simulink model "SRRC_Cosimulation"  (R2016a)
settings: Solver=ode3  StartTime=0.0  StopTime=0.5  RelTol=1e-3
undefined symbols (not defined in the file or in its folder): image, port_label
libraries: aldec_ahdl x2, dspsrcs4 x2
settings Model: Creator=Sara  LastModifiedBy=paolosassi
settings DataIOCC: LimitDataPoints=on  SaveFormat=Array
settings HardwareCC: ProdBitPerPointer=32  ProdLargestAtomicFloat=None  ProdIntDivRoundTo=Undefined  ProdEndianess=Unspecified  ProdWordSize=32  ProdHWDeviceType=32-bit Generic
settings ModelReferenceCC: PropagateSignalLabelsOutOfModel=off
settings ConfigComp: CovModelRefEnable=Off

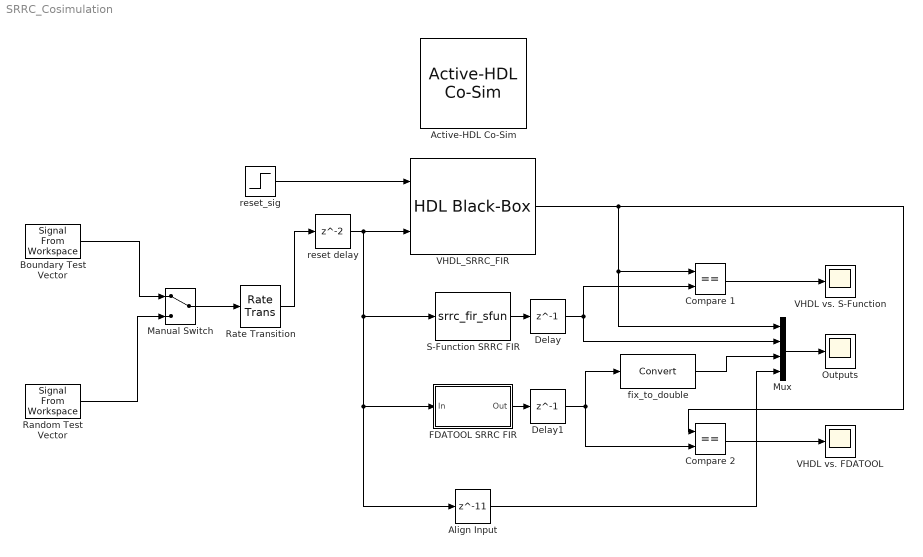
== system SRRC_Cosimulation ==
  Active-HDL Co-Sim : aldec_ahdl/Active-HDL Co-Sim  Tag=Active-HDL_Co-Sim_close  hdl_period=8  hdl_tscale=ms  sys_period=[500, 0]  sys_tscale=As In Simulator  wav_fn=$(model_name)  wav_settings=[0,0,0,0,0,0,0,0]  dbg=off  auto_start=off  gen_tb=[0,1,15]  batch_sim=off  tb_fn=mlab_post_tb.log  metavalue_map=[0,0]  sim_resolution=[1,0,0]  active_page=1  aws_en=on  aws_file=C:\Users\Sara\Desktop\Corsi\Digital Systems Design\Project\DSS_Project\DSS_Project.aws  ahdl_en=off  blk_ver=10.3.RTM  macro_en=[0,0,0]
  Align Input : Delay  DelayLength=11
  Boundary Test Vector : dspsrcs4/Signal From Workspace  X=bt_tv  Ts=0.032  nsamps=1  OutputAfterFinalValue=Setting to zero  ignoreOrWarnInputAndFrameLengths=off  OutputFrames=on
  Compare 1 : RelationalOperator  Operator===  OutDataTypeStr=boolean
  Compare 2 : RelationalOperator  Operator===  OutDataTypeStr=boolean
  Delay : Delay  DelayLength=1
  Delay1 : Delay  DelayLength=1
  FDATOOL SRRC FIR : Subsystem  Tag=BlockMethodSubSystem
  Manual Switch : ManualSwitch
  Mux : Mux
  Outputs : Scope
  Random Test Vector : dspsrcs4/Signal From Workspace  X=rand_tv  Ts=0.032  nsamps=1  OutputAfterFinalValue=Setting to zero  ignoreOrWarnInputAndFrameLengths=off  OutputFrames=on
  Rate Transition : RateTransition
  S-Function SRRC FIR : M-S-Function  FunctionName=srrc_fir_sfun
  VHDL vs. FDATOOL : Scope
  VHDL vs. S-Function : Scope
  VHDL_SRRC_FIR : aldec_ahdl/HDL Black-Box  Tag=Active-HDL_BB_lib  module_m=fir_srrc  ports_cfg={clk,3,1,2,0,1,8,0,0,1,0,1}{reset,0,1,2,0,clk,8,0,0,0,0,1}{x,0,16,2,0,clk,0,1,0,0,0,1}{y,1,19,2,0,1,0,0,0,0,0,1}  clocks={0,1,0,0.5,0}  waves={0,clk,0,0,0,15,,-1,-1,-1,0,0,0,0}{0,x,2,2,0,100,,-1,-1,-1,1,0,0,0}{0,y,2,2,0,100,,-1,-1,-1,1,0,0,0}{0,reset,0,0,0,15,,-1,-1,-1,0,0,0,0}  block_mask=image('HDLBlackBox.jpg','center'); disp('fir_srrc');port_label('input', 1, 'reset');port_label('input', 2, 'x');port_label('output', 1, 'y');  config=[2,1]  inp=[2, 8, 1, 0, 0, 0, 2, 0, 16, 0, 1, 0, 2]  out=[1, 0, 19, 0, 0, 0, 2]  sampling=[1, 1, 1, 1]  active_page={0}{80,0,35,1,65,2,70,3,70,4,60,5,60,6,50,7,35,8,35,9,119,10}{103,0,55,1,70,2,75,3,75,4,45,5,45,6,45,7,165,8,0,0,0,0}{165,0,130,1,190,2,190,3,0,0,0,0,0,0,0,0,0,0,0,0,0,0}{81,0,60,1,60,2,70,3,60,4,0,0,0,0,0,0,0,0,0,0,0,0}{83,0,70,1,80,2,50,3,50,4,0,0,0,0,0,0,0,0,0,0,0,0}{125,0,330,1,220,2,0,0,0,0,0,0,0,0,0,0,0,0,0,0,0,0}{95,0,95,1,70,2,50,3,80,4,35,5,35,6,65,7,150,8,0,0,0,0}{766,476}  param_val=0  clk_val=[1,0,0.5]  ce_val=[0]  blk_ver=10.3.RTM  blk_conf=0  user_conv=0
  fix_to_double : DataTypeConversion
  reset delay : Delay
  reset_sig : Step  Time=0.01  Before=1  After=0  SampleTime=0
  wires:
  reset_sig/1 -> VHDL_SRRC_FIR/1
  VHDL_SRRC_FIR/1 -> Compare 2/1, Mux/1, Compare 1/1
  Random Test Vector/1 -> Manual Switch/2
  Rate Transition/1 -> reset delay/1
  reset delay/1 -> VHDL_SRRC_FIR/2, S-Function SRRC FIR/1, Align Input/1, FDATOOL SRRC FIR/1(In)
  FDATOOL SRRC FIR/1(Out) -> Delay1/1
  Compare 1/1 -> VHDL vs. S-Function/1
  S-Function SRRC FIR/1 -> Delay/1
  Manual Switch/1 -> Rate Transition/1
  Boundary Test Vector/1 -> Manual Switch/1
  Compare 2/1 -> VHDL vs. FDATOOL/1
  Align Input/1 -> Mux/4
  Mux/1 -> Outputs/1
  fix_to_double/1 -> Mux/3
  Delay/1 -> Mux/2, Compare 1/2
  Delay1/1 -> Compare 2/2, fix_to_double/1

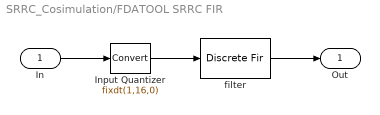
== system SRRC_Cosimulation/FDATOOL SRRC FIR ==
  In : Inport
  Input Quantizer : DataTypeConversion  OutDataTypeStr=fixdt(1,16,0)  RndMeth=Round  SaturateOnIntegerOverflow=on
  filter : DiscreteFir  Coefficients=[-0.016500000000000001 -0.014999999999999999 0.0155 0.0424 0.0155 -0.074999999999999997 -0.15679999999999999 -0.1061 0.15679999999999999 0.5786 0.97450000000000003 1.1366000000000001 0.97450000000000003 0.5786 0.15679999999999999 -0.1061 -0.15679999999999999 -0.074999999999999997 0.0155 0.0424 0.0155 -0.014999999999999999 -0.016500000000000001]  CoefDataTypeStr=fixdt(true,16,14)  ProductDataTypeStr=fixdt(true,32,0)  AccumDataTypeStr=fixdt(true,33,0)  OutDataTypeStr=fixdt(true,19,0)
  Out : Outport
  wires:
  In/1 -> Input Quantizer/1
  Input Quantizer/1 -> filter/1
  filter/1 -> Out/1
